simulink model "F16_model_propulsion_og"  (R2025b)
settings: Solver=VariableStepAuto  StartTime=0.0  StopTime=10.0  RelTol=1e-3
values from neighbouring files (symbols this model uses):
  b = 9.144    [initialization.m]
  c_bar = 3.45    [initialization.m]
  g = 9.81    [initialization.m]
  I = [Ixx 0 -Ixz; 0 Iyy 0; -Ixz 0 Izz]    [initialization.m]
  S = 27.87    [initialization.m]
  xcg = 0.3*c_bar    (= 1.035)    [initialization.m]
  xcgr = 0.35*c_bar    (= 1.2075)    [initialization.m]
undefined symbols (not defined in the file or in its folder): aero_data
libraries: simulink_extras x2, matrix_library x2
(part 1 of 2)
settings Model: Creator=deepa  LastModifiedBy=deepa

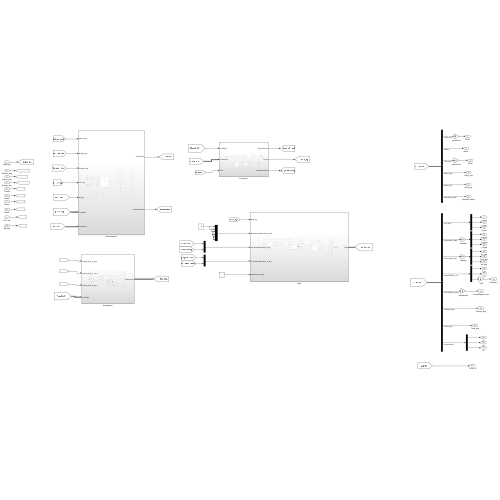
[thumbnail: Simulink's stored preview of the top-level diagram]
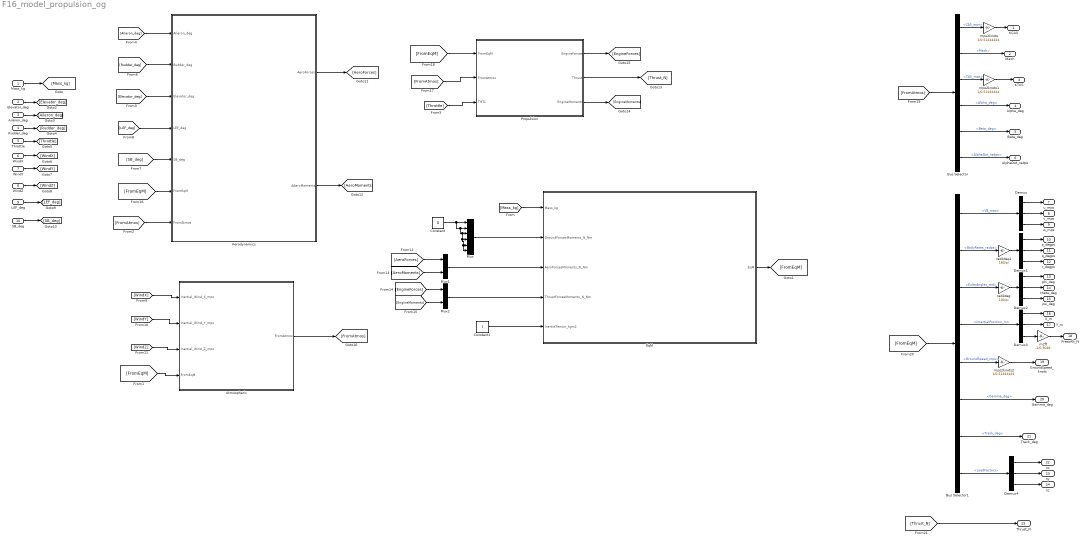
== system F16_model_propulsion_og ==
  Mass_kg : Inport  OutDataTypeStr=double
  Elevator_deg : Inport  Port=2  OutDataTypeStr=double
  Aileron_deg : Inport  Port=3  OutDataTypeStr=double
  Rudder_deg : Inport  Port=4  OutDataTypeStr=double
  Throttle : Inport  Port=5  OutDataTypeStr=double
  WindX : Inport  Port=6  OutDataTypeStr=double
  WindY : Inport  Port=7  OutDataTypeStr=double
  WindZ : Inport  Port=8  OutDataTypeStr=double
  LEF_deg : Inport  Port=9
  SB_deg : Inport  Port=10
  Aerodynamics : Subsystem
  Atmospheric : Subsystem
  Bus Selector : BusSelector  OutputSignals=CAS_mps,Mach,TAS_mps,Alpha_deg,Beta_deg,AlphaDot_radps
  Bus Selector1 : BusSelector  OutputSignals=VB_mps,BodyRates_radps,EulerAngles_rad,IntertialPosition_m,GroundSpeed_mps,Gamma_deg,Track_deg,LoadFactors
  Constant : Constant  Value=0
  Constant1 : Constant  Value=I
  Demux{,1..4} (5 alike) : Demux  Outputs=3
  EqM : Subsystem
  Mux : Mux  Inputs=6
  Mux1 : Mux  Inputs=2
  Mux2 : Mux  Inputs=2
  Propulsion : Subsystem
  m2ft : Gain  Gain=-1/0.3048
  mps2knots : Gain  Gain=1/0.51444444
  mps2knots1 : Gain  Gain=1/0.51444444
  mps2knots2 : Gain  Gain=1/0.51444444
  rad2deg : Gain  Gain=180/pi
  rad2deg1 : Gain  Gain=180/pi
  KCAS : Outport
  Mach : Outport  Port=2
  KTAS : Outport  Port=3
  Alpha_deg : Outport  Port=4
  Beta_deg : Outport  Port=5
  AlphaDot_radps : Outport  Port=6
  u_mps : Outport  Port=7
  v_mps : Outport  Port=8
  w_mps : Outport  Port=9
  p_degps : Outport  Port=10
  q_degps : Outport  Port=11
  r_degps : Outport  Port=12
  phi_deg : Outport  Port=13
  theta_deg : Outport  Port=14
  psi_deg : Outport  Port=15
  X_m : Outport  Port=16
  Y_m : Outport  Port=17
  PressAlt_ft : Outport  Port=18
  GroundSpeed_knots : Outport  Port=19
  Gamma_deg : Outport  Port=20
  Track_deg : Outport  Port=21
  nx : Outport  Port=22
  ny : Outport  Port=23
  nz : Outport  Port=24
  Thrust_N : Outport  Port=25
  wires:
  [FromAtmos] -> Propulsion/2(FromAtmos)
  Propulsion/2(Thrust) -> [Thrust_N]
  Mux/1 -> EqM/2(GroundForcesMoments_N_Nm)
  [FromEqM] -> Bus Selector1/1
  [EngineForces] -> Mux2/1
  Demux/3 -> w_mps/1
  Demux2/1 -> phi_deg/1
  [WindZ] -> Atmospheric/3(Inertial_Wind_Z_mps)
  Bus Selector1/3 -> rad2deg/1  "<EulerAngles_rad>"
  Demux1/3 -> r_degps/1
  [AeroMoments] -> Mux1/2
  LEF_deg/1 -> [LEF_deg]
  Mass_kg/1 -> [Mass_kg]
  Bus Selector1/5 -> mps2knots2/1  "<GroundSpeed_mps>"
  Bus Selector/2 -> Mach/1  "<Mach>"
  EqM/1(EqM) -> [FromEqM]
  rad2deg/1 -> Demux2/1
  Bus Selector/6 -> AlphaDot_radps/1  "<AlphaDot_radps>"
  Demux3/1 -> X_m/1
  [FromAtmos] -> Aerodynamics/7(FromAtmos)
  [Thrust_N] -> Thrust_N/1
  Demux2/3 -> psi_deg/1
  Throttle/1 -> [Throttle]
  Demux2/2 -> theta_deg/1
  Demux3/2 -> Y_m/1
  [EngineMoments] -> Mux2/2
  Demux4/2 -> ny/1
  Demux/2 -> v_mps/1
  Demux/1 -> u_mps/1
  Bus Selector/4 -> Alpha_deg/1  "<Alpha_deg>"
  [AeroForces] -> Mux1/1
  Demux4/3 -> nz/1
  [Rudder_deg] -> Aerodynamics/2(Rudder_deg)
  Elevator_deg/1 -> [Elevator_deg]
  Atmospheric/1(FromAtmos) -> [FromAtmos]
  Aerodynamics/2(AAeroMoments) -> [AeroMoments]
  Bus Selector/1 -> mps2knots/1  "<CAS_mps>"
  mps2knots/1 -> KCAS/1
  WindZ/1 -> [WindZ]
  Demux1/1 -> p_degps/1
  [SB_deg] -> Aerodynamics/5(SB_deg)
  rad2deg1/1 -> Demux1/1
  [FromAtmos] -> Bus Selector/1
  [FromEqM] -> Aerodynamics/6(FromEqM)
  [LEF_deg] -> Aerodynamics/4(LEF_deg)
  [Mass_kg] -> EqM/1(Mass_kg)
  WindX/1 -> [WindX]
  [WindX] -> Atmospheric/1(Inertial_Wind_X_mps)
  Demux4/1 -> nx/1
  Mux1/1 -> EqM/3(AeroForcesMoments_N_Nm)
  Bus Selector1/8 -> Demux4/1  "<LoadFactors>"
  mps2knots2/1 -> GroundSpeed_knots/1
  m2ft/1 -> PressAlt_ft/1
  Constant/1 -> Mux/1, Mux/6, Mux/5, Mux/4, Mux/3, Mux/2
  [Aileron_deg] -> Aerodynamics/1(Aileron_deg)
  Bus Selector1/4 -> Demux3/1  "<IntertialPosition_m>"
  Bus Selector1/7 -> Track_deg/1  "<Track_deg>"
  Mux2/1 -> EqM/4(ThrustForcesMoments_N_Nm)
  Demux1/2 -> q_degps/1
  Demux3/3 -> m2ft/1
  Constant1/1 -> EqM/5(InertiaTensor_kgm2)
  Bus Selector1/2 -> rad2deg1/1  "<BodyRates_radps>"
  Rudder_deg/1 -> [Rudder_deg]
  [WindY] -> Atmospheric/2(Inertial_Wind_Y_mps)
  Aileron_deg/1 -> [Aileron_deg]
  [Elevator_deg] -> Aerodynamics/3(Elevator_deg)
  Bus Selector/5 -> Beta_deg/1  "<Beta_deg>"
  Bus Selector/3 -> mps2knots1/1  "<TAS_mps>"
  SB_deg/1 -> [SB_deg]
  Bus Selector1/1 -> Demux/1  "<VB_mps>"
  Aerodynamics/1(AeroForces) -> [AeroForces]
  WindY/1 -> [WindY]
  [FromEqM] -> Atmospheric/4(FromEqM)
  Bus Selector1/6 -> Gamma_deg/1  "<Gamma_deg>"
  mps2knots1/1 -> KTAS/1
  [Throttle] -> Propulsion/3(THTL)
  [FromEqM] -> Propulsion/1(FromEqM)
  Propulsion/1(EngineForces) -> [EngineForces]
  Propulsion/3(EngineMoments) -> [EngineMoments]

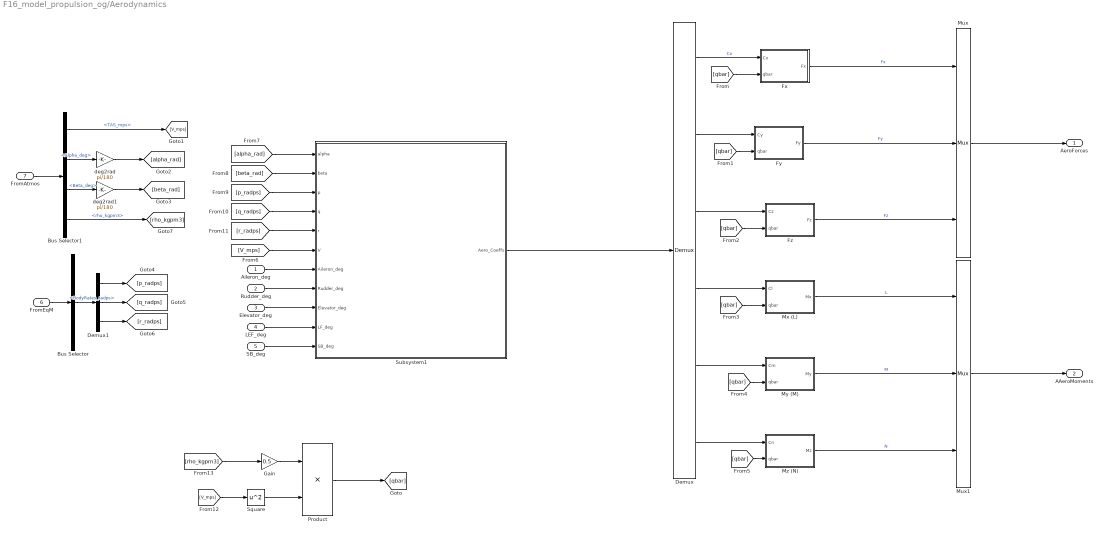
== system F16_model_propulsion_og/Aerodynamics ==
  Aileron_deg : Inport
  Rudder_deg : Inport  Port=2
  Elevator_deg : Inport  Port=3
  LEF_deg : Inport  Port=4
  SB_deg : Inport  Port=5
  FromEqM : Inport  Port=6
  FromAtmos : Inport  Port=7
  Bus Selector : BusSelector  OutputSignals=BodyRates_radps
  Bus Selector1 : BusSelector  OutputSignals=TAS_mps,Alpha_deg,Beta_deg,rho_kgpm3
  Demux : Demux  Outputs=6
  Demux1 : Demux  Outputs=3
  Fx : Subsystem
  Fy : Subsystem
  Fz : Subsystem
  Gain : Gain  Gain=0.5
  Mux : Mux  Inputs=3
  Mux1 : Mux  Inputs=3
  Mx (L) : Subsystem
  My (M) : Subsystem
  Mz (N) : Subsystem
  Product : Product
  Square : Math  Operator=square
  Subsystem1 : Subsystem
  deg2rad : Gain  Gain=pi/180
  deg2rad1 : Gain  Gain=pi/180
  AeroForces : Outport
  AAeroMoments : Outport  Port=2
  wires:
  [qbar] -> Mz (N)/2(qbar)
  Fx/1(Fx) -> Mux/1  "Fx"
  My (M)/1(My) -> Mux1/2  "M"
  [qbar] -> Fz/2(qbar)
  Fy/1(Fy) -> Mux/2  "Fy"
  Aileron_deg/1 -> Subsystem1/7(Aileron_deg)
  [qbar] -> Fx/2(qbar)
  Mux/1 -> AeroForces/1
  Subsystem1/1(Aero_Coeffs) -> Demux/1
  Fz/1(Fz) -> Mux/3  "Fz"
  [qbar] -> Fy/2(qbar)
  Demux/2 -> Fy/1(Cy)
  [p_radps] -> Subsystem1/3(p)
  [beta_rad] -> Subsystem1/2(beta)
  Demux/1 -> Fx/1(Cx)  "Cx"
  [V_mps] -> Subsystem1/6(V)
  [qbar] -> Mx (L)/2(qbar)
  [qbar] -> My (M)/2(qbar)
  Demux/4 -> Mx (L)/1(Cl)
  [alpha_rad] -> Subsystem1/1(alpha)
  Demux/6 -> Mz (N)/1(Cn)
  Demux/5 -> My (M)/1(Cm)
  Mz (N)/1(Mz) -> Mux1/3  "N"
  Mx (L)/1(Mx) -> Mux1/1  "L"
  Demux/3 -> Fz/1(Cz)
  Mux1/1 -> AAeroMoments/1
  [r_radps] -> Subsystem1/5(r)
  [q_radps] -> Subsystem1/4(q)
  Rudder_deg/1 -> Subsystem1/8(Rudder_deg)
  SB_deg/1 -> Subsystem1/11(SB_deg)
  LEF_deg/1 -> Subsystem1/10(LF_deg)
  Elevator_deg/1 -> Subsystem1/9(Elevator_deg)
  FromEqM/1 -> Bus Selector/1
  FromAtmos/1 -> Bus Selector1/1
  Bus Selector1/1 -> [V_mps]  "<TAS_mps>"
  Bus Selector1/2 -> deg2rad/1  "<Alpha_deg>"
  Bus Selector1/3 -> deg2rad1/1  "<Beta_deg>"
  deg2rad/1 -> [alpha_rad]
  deg2rad1/1 -> [beta_rad]
  Bus Selector/1 -> Demux1/1  "<BodyRates_radps>"
  Demux1/1 -> [p_radps]
  Demux1/2 -> [q_radps]
  Demux1/3 -> [r_radps]
  Bus Selector1/4 -> [rho_kgpm3]  "<rho_kgpm3>"
  [V_mps] -> Square/1
  Square/1 -> Product/2
  [rho_kgpm3] -> Gain/1
  Gain/1 -> Product/1
  Product/1 -> [qbar]

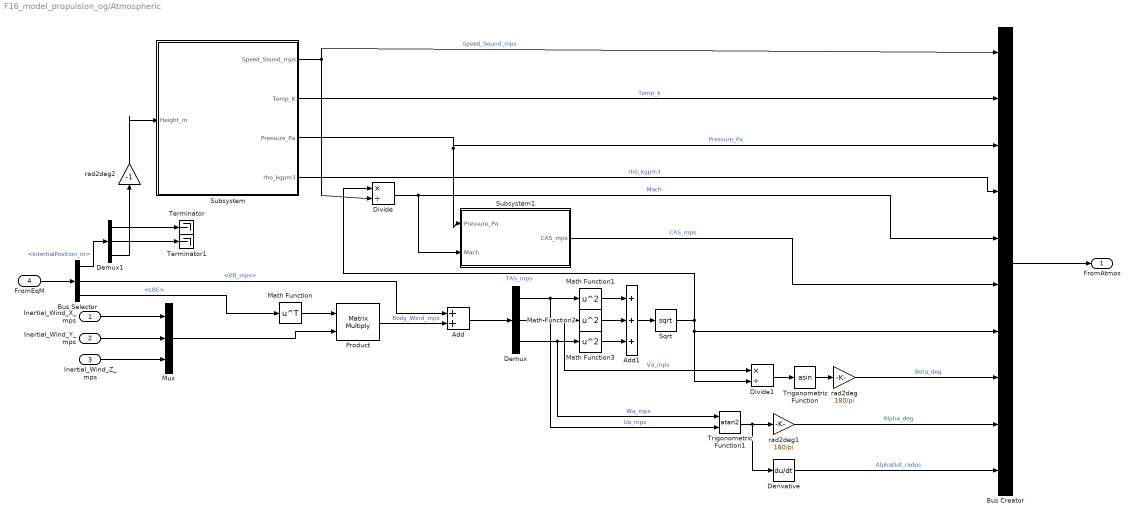
== system F16_model_propulsion_og/Atmospheric ==
  Inertial_Wind_X_mps : Inport
  Inertial_Wind_Y_mps : Inport  Port=2
  Inertial_Wind_Z_mps : Inport  Port=3
  FromEqM : Inport  Port=4
  Add : Sum
  Add1 : Sum  Inputs=+++
  Bus Creator : BusCreator  Inputs=10
  Bus Selector : BusSelector  OutputSignals=IntertialPosition_m,VB_mps,LBE
  Demux : Demux  Outputs=3
  Demux1 : Demux  Outputs=3
  Derivative : Derivative
  Divide : Product  Inputs=*/
  Divide1 : Product  Inputs=*/
  Math Function : Math  Operator=transpose  SignedPower=on
  Math Function1 : Math  Operator=square  SignedPower=on
  Math Function2 : Math  Operator=square  SignedPower=on
  Math Function3 : Math  Operator=square  SignedPower=on
  Mux : Mux  Inputs=3
  Product : Product  Multiplication=Matrix(*)
  Sqrt : Sqrt
  Subsystem : Subsystem
  Subsystem1 : Subsystem
  Terminator : Terminator
  Terminator1 : Terminator
  Trigonometric Function : Trigonometry  Operator=asin
  Trigonometric Function1 : Trigonometry  Operator=atan2
  rad2deg : Gain  Gain=180/pi
  rad2deg1 : Gain  Gain=180/pi
  rad2deg2 : Gain  Gain=-1
  FromAtmos : Outport
  wires:
  Inertial_Wind_Y_mps/1 -> Mux/2
  Demux/3 -> Math Function3/1, Trigonometric Function1/1  "Wa_mps"
  Bus Selector/1 -> Demux1/1  "<IntertialPosition_m>"
  Mux/1 -> Product/2
  Demux/1 -> Math Function1/1, Trigonometric Function1/2  "Ua_mps"
  rad2deg1/1 -> Bus Creator/9  "Alpha_deg"
  Subsystem/2(Temp_K) -> Bus Creator/2  "Temp_k"
  Bus Selector/3 -> Math Function/1  "<LBE>"
  Trigonometric Function/1 -> rad2deg/1
  rad2deg/1 -> Bus Creator/8  "Beta_deg"
  Subsystem/4(rho_kgpm3) -> Bus Creator/4  "rho_kgpm3"
  Bus Creator/1 -> FromAtmos/1
  Subsystem/3(Pressure_Pa) -> Subsystem1/1(Pressure_Pa), Bus Creator/3  "Pressure_Pa"
  Demux/2 -> Math Function2/1, Divide1/1  "Va_mps"
  Subsystem1/1(CAS_mps) -> Bus Creator/6  "CAS_mps"
  Demux1/2 -> Terminator1/1
  Divide1/1 -> Trigonometric Function/1
  Subsystem/1(Speed_Sound_mps) -> Divide/2, Bus Creator/1  "Speed_Sound_mps"
  Divide/1 -> Subsystem1/2(Mach), Bus Creator/5  "Mach"
  Demux1/1 -> Terminator/1
  Math Function2/1 -> Add1/2
  Add/1 -> Demux/1
  Derivative/1 -> Bus Creator/10  "AlphaDot_radps"
  Math Function/1 -> Product/1
  Math Function1/1 -> Add1/1
  Bus Selector/2 -> Add/1  "<VB_mps>"
  Inertial_Wind_X_mps/1 -> Mux/1
  Sqrt/1 -> Divide/1, Bus Creator/7, Divide1/2  "TAS_mps"
  FromEqM/1 -> Bus Selector/1
  Trigonometric Function1/1 -> rad2deg1/1, Derivative/1
  Inertial_Wind_Z_mps/1 -> Mux/3
  Product/1 -> Add/2  "Body_Wind_mps"
  rad2deg2/1 -> Subsystem/1("Height_m ")
  Demux1/3 -> rad2deg2/1
  Add1/1 -> Sqrt/1
  Math Function3/1 -> Add1/3

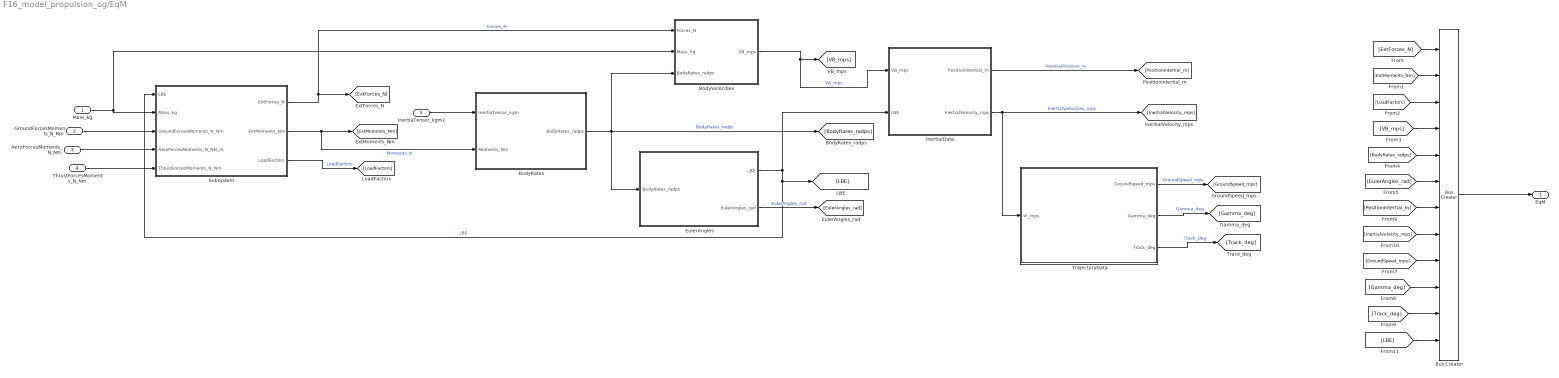
== system F16_model_propulsion_og/EqM ==
  Mass_kg : Inport
  GroundForcesMoments_N_Nm : Inport  Port=2
  AeroForcesMoments_N_Nm : Inport  Port=3
  ThrustForcesMoments_N_Nm : Inport  Port=4
  InertiaTensor_kgm2 : Inport  Port=5
  BodyRates : Subsystem
  BodyVelocities : Subsystem
  Bus Creator : BusCreator  Inputs=12
  EulerAngles : Subsystem
  InertialData : Subsystem
  Subsystem : Subsystem
  TrajectoryData : Subsystem
  EqM : Outport
  wires:
  InertiaTensor_kgm2/1 -> BodyRates/1(InertiaTensor_kgm)
  BodyRates/1(BodyRates_radps) -> EulerAngles/1(BodyRates_radps), BodyVelocities/3(BodyRates_radps), [BodyRates_radps]  "BodyRates_radps"
  AeroForcesMoments_N_Nm/1 -> Subsystem/4(AeroForcesMoments_N_NN_m)
  InertialData/1(PositionIntertial_m) -> [PositionIntertial_m]  "IntertialPosition_m"
  [GroundSpeed_mps] -> Bus Creator/9
  [PositionIntertial_m] -> Bus Creator/7
  TrajectoryData/1(GroundSpeed_mps) -> [GroundSpeed_mps]  "GroundSpeed_mps"
  Subsystem/2(ExtMoments_Nm) -> BodyRates/2(Moments_Nm), [ExtMoments_Nm]  "Moments_N"
  InertialData/2(InertialVelocity_mps) -> TrajectoryData/1(VI_mps), [InertialVelocity_mps]  "InertialVelocities_mps"
  [Track_deg] -> Bus Creator/11
  Subsystem/1(ExtForces_N) -> BodyVelocities/1(Forces_N), [ExtForces_N]  "Forces_N"
  [VB_mps] -> Bus Creator/4
  [LoadFactors] -> Bus Creator/3
  BodyVelocities/1(VB_mps) -> InertialData/1(VB_mps), [VB_mps]  "VB_mps"
  EulerAngles/2(EulerAngles_rad) -> [EulerAngles_rad]  "EulerAngles_rad"
  TrajectoryData/3(Track_deg) -> [Track_deg]  "Track_deg"
  EulerAngles/1(LBE) -> InertialData/2(LBE), Subsystem/1(LBE), [LBE]  "LBE"
  TrajectoryData/2(Gamma_deg) -> [Gamma_deg]  "Gamma_deg"
  [BodyRates_radps] -> Bus Creator/5
  [Gamma_deg] -> Bus Creator/10
  [LBE] -> Bus Creator/12
  Subsystem/3(LoadFactors) -> [LoadFactors]  "LoadFactors"
  [EulerAngles_rad] -> Bus Creator/6
  [InertialVelocity_mps] -> Bus Creator/8
  ThrustForcesMoments_N_Nm/1 -> Subsystem/5(ThrustForcesMoments_N_Nm)
  GroundForcesMoments_N_Nm/1 -> Subsystem/3(GroundForcesMoments_N_Nm)
  Bus Creator/1 -> EqM/1
  [ExtMoments_Nm] -> Bus Creator/2
  [ExtForces_N] -> Bus Creator/1
  Mass_kg/1 -> BodyVelocities/2(Mass_kg), Subsystem/2(Mass_kg)

== system F16_model_propulsion_og/Propulsion ==
  FromEqM : Inport
  FromAtmos : Inport  Port=2
  THTL : Inport  Port=3
  Bus Selector : BusSelector  OutputSignals=IntertialPosition_m
  Bus Selector1 : BusSelector  OutputSignals=Mach
  Gain : Gain  Gain=-1
  Integrator : Integrator  ContinuousStateAttributes='POW'
  Mux : Mux  Inputs=3
  Mux1 : Mux  Inputs=3
  PDOT : MATLAB Function  TreatAsAtomicUnit=on
  Selector : Selector  InputPortWidth=3  IndexOptions=Index vector (dialog)  Indices=[3]  OutputSizes=1
  TGEAR : MATLAB Function  TreatAsAtomicUnit=on
  Thrust_ : MATLAB Function  TreatAsAtomicUnit=on
  Zero : Constant  Value=0  OutDataTypeStr=Inherit: Inherit via back propagation
  Zero1 : Constant  Value=0  OutDataTypeStr=Inherit: Inherit via back propagation
  EngineForces : Outport
  Thrust : Outport  Port=2
  EngineMoments : Outport  Port=3
  wires:
  FromEqM/1 -> Bus Selector/1
  TGEAR/1(TGEAR) -> PDOT/2(P1)
  THTL/1 -> TGEAR/1(THTL)
  Mux/1 -> EngineMoments/1
  Bus Selector1/1 -> Thrust_/3(MACH)  "<Mach>"
  Thrust_/1(THRUST) -> Thrust/1, Mux1/1
  Gain/1 -> Thrust_/2(ALT)
  FromAtmos/1 -> Bus Selector1/1
  Bus Selector/1 -> Selector/1  "<IntertialPosition_m>"
  Zero/1 -> Mux/1, Mux/3, Mux/2
  Mux1/1 -> EngineForces/1
  PDOT/1(PDOT) -> Integrator/1  "Pdot"
  Zero1/1 -> Mux1/2, Mux1/3
  Integrator/1 -> PDOT/1(P3), Thrust_/1(POW)
  Selector/1 -> Gain/1

== system F16_model_propulsion_og/Aerodynamics/Fx ==
  Cx : Inport
  qbar : Inport  Port=2
  Gain : Gain  Gain=S
  Product : Product
  Fx : Outport
  wires:
  Product/1 -> Fx/1
  Gain/1 -> Product/1
  qbar/1 -> Product/2
  Cx/1 -> Gain/1

== system F16_model_propulsion_og/Aerodynamics/Fy ==
  Cy : Inport
  qbar : Inport  Port=2
  Gain : Gain  Gain=S
  Product : Product
  Fy : Outport
  wires:
  Cy/1 -> Gain/1
  qbar/1 -> Product/2
  Gain/1 -> Product/1
  Product/1 -> Fy/1

== system F16_model_propulsion_og/Aerodynamics/Fz ==
  Cz : Inport
  qbar : Inport  Port=2
  Gain : Gain  Gain=S
  Product : Product
  Fz : Outport
  wires:
  Product/1 -> Fz/1
  Gain/1 -> Product/1
  qbar/1 -> Product/2
  Cz/1 -> Gain/1

== system F16_model_propulsion_og/Aerodynamics/Mx (L) ==
  Cl : Inport
  qbar : Inport  Port=2
  Gain : Gain  Gain=S*b
  Product : Product
  Mx : Outport
  wires:
  Cl/1 -> Gain/1
  qbar/1 -> Product/2
  Gain/1 -> Product/1
  Product/1 -> Mx/1

== system F16_model_propulsion_og/Aerodynamics/My (M) ==
  Cm : Inport
  qbar : Inport  Port=2
  Gain : Gain  Gain=S*c_bar
  Product : Product
  My : Outport
  wires:
  Product/1 -> My/1
  Gain/1 -> Product/1
  qbar/1 -> Product/2
  Cm/1 -> Gain/1

== system F16_model_propulsion_og/Aerodynamics/Mz (N) ==
  Cn : Inport
  qbar : Inport  Port=2
  Gain : Gain  Gain=S*b
  Product : Product
  Mz : Outport
  wires:
  Cn/1 -> Gain/1
  qbar/1 -> Product/2
  Gain/1 -> Product/1
  Product/1 -> Mz/1

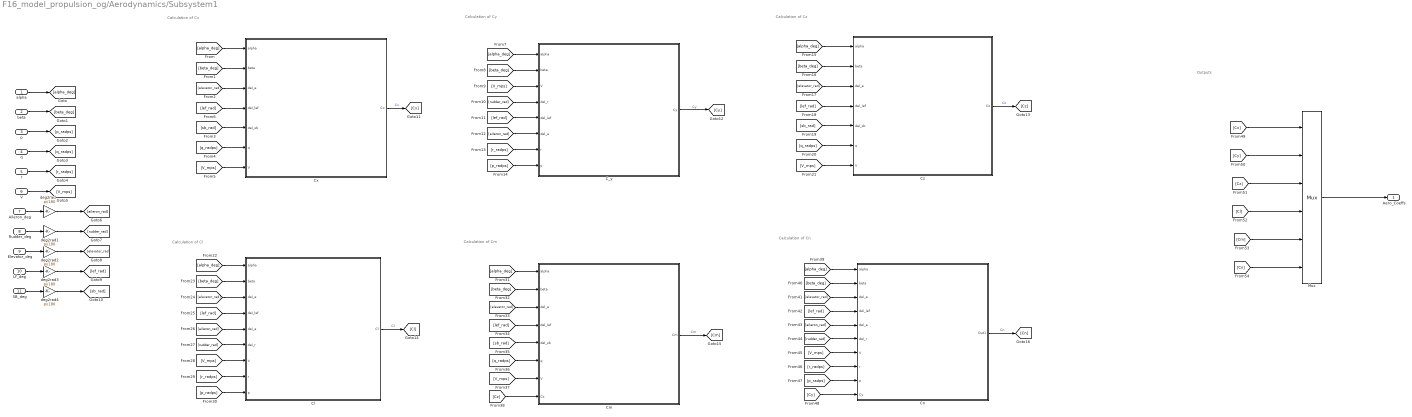
== system F16_model_propulsion_og/Aerodynamics/Subsystem1 ==
  note: Calculation of Cm
  note: Outputs
  note: Calculation of Cz
  note: Calculation of Cy
  note: Calculation of Cx
  note: Calculation of Cl
  note: Calculation of Cn
  alpha : Inport
  beta : Inport  Port=2
  p : Inport  Port=3
  q : Inport  Port=4
  r : Inport  Port=5
  V : Inport  Port=6
  Aileron_deg : Inport  Port=7
  Rudder_deg : Inport  Port=8
  Elevator_deg : Inport  Port=9
  LF_deg : Inport  Port=10
  SB_deg : Inport  Port=11
  C_y : Subsystem
  Cl : Subsystem
  Cm : Subsystem
  Cn : Subsystem
  Cx : Subsystem
  Cz : Subsystem
  Mux : Mux  Inputs=6
  deg2rad{,1..4} (5 alike) : Gain  Gain=pi/180
  Aero_Coeffs : Outport
  wires:
  V/1 -> [V_mps]
  [lef_rad] -> C_y/5(del_lef)
  [Cz] -> Mux/3
  [alpha_deg] -> C_y/1(alpha)
  [q_radps] -> Cx/6(q)
  [V_mps] -> C_y/3(V)
  alpha/1 -> [alpha_deg]
  [elevator_rad] -> Cm/3(del_e)
  Cx/1(Cx) -> [Cx]  "Cx"
  [elevator_rad] -> Cz/3(del_e)
  [rudder_rad] -> Cn/6(del_r)
  [r_radps] -> Cn/8(r)
  [beta_deg] -> C_y/2(beta)
  [elevator_rad] -> Cx/3(del_e)
  [lef_rad] -> Cx/4(del_lef)
  [Cl] -> Mux/4
  [alpha_deg] -> Cx/1(alpha)
  [alpha_deg] -> Cn/1(alpha)
  [p_radps] -> Cn/9(p)
  r/1 -> [r_radps]
  Cl/1(Cl) -> [Cl]  "Cl"
  C_y/1(Cy) -> [Cy]  "Cy"
  Cz/1(Cz) -> [Cz]  "Cz"
  [r_radps] -> Cl/8(r)
  SB_deg/1 -> deg2rad4/1
  LF_deg/1 -> deg2rad3/1
  [elevator_rad] -> Cn/3(del_e)
  [beta_deg] -> Cm/2(beta)
  [p_radps] -> C_y/8(p)
  [q_radps] -> Cm/6(q)
  [alpha_deg] -> Cz/1(alpha)
  [V_mps] -> Cl/7(V)
  [alpha_deg] -> Cl/1(alpha)
  [beta_deg] -> Cl/2(beta)
  [lef_rad] -> Cz/4(del_lef)
  Mux/1 -> Aero_Coeffs/1
  [alpha_deg] -> Cm/1(alpha)
  [V_mps] -> Cm/7(V)
  beta/1 -> [beta_deg]
  Rudder_deg/1 -> deg2rad1/1
  [sb_rad] -> Cz/5(del_sb)
  [sb_rad] -> Cx/5(del_sb)
  [Cy] -> Mux/2
  [rudder_rad] -> C_y/4(del_r)
  Aileron_deg/1 -> deg2rad/1
  [beta_deg] -> Cz/2(beta)
  [Cz] -> Cm/8(Cz)
  [V_mps] -> Cz/7(V)
  [V_mps] -> Cn/7(V)
  [r_radps] -> C_y/7(r)
  [lef_rad] -> Cl/4(del_lef)
  [sb_rad] -> Cm/5(del_sb)
  [q_radps] -> Cz/6(q)
  [Cm] -> Mux/5
  Elevator_deg/1 -> deg2rad2/1
  q/1 -> [q_radps]
  [aileron_rad] -> Cn/5(del_a)
  [p_radps] -> Cl/9(p)
  [rudder_rad] -> Cl/6(del_r)
  [elevator_rad] -> Cl/3(del_e)
  p/1 -> [p_radps]
  [aileron_rad] -> Cl/5(del_a)
  [Cn] -> Mux/6
  [lef_rad] -> Cm/4(del_lef)
  [beta_deg] -> Cn/2(beta)
  [Cy] -> Cn/10(Cy)
  [aileron_rad] -> C_y/6(del_a)
  [V_mps] -> Cx/7(V)
  Cn/1(Out1) -> [Cn]  "Cn"
  [beta_deg] -> Cx/2(beta)
  [lef_rad] -> Cn/4(del_lef)
  [Cx] -> Mux/1
  Cm/1(Cm) -> [Cm]  "Cm"
  deg2rad/1 -> [aileron_rad]
  deg2rad1/1 -> [rudder_rad]
  deg2rad2/1 -> [elevator_rad]
  deg2rad3/1 -> [lef_rad]
  deg2rad4/1 -> [sb_rad]

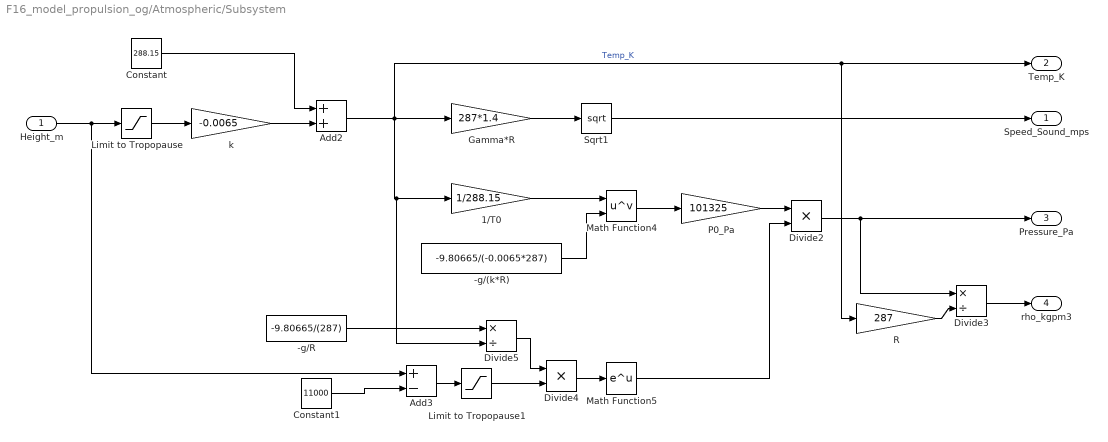
== system F16_model_propulsion_og/Atmospheric/Subsystem ==
  "Height_m " : Inport
  -g/(k*R) : Constant  Value=-9.80665/(-0.0065*287)
  -g/R : Constant  Value=-9.80665/(287)
  1/T0 : Gain  Gain=1/288.15
  Add2 : Sum
  Add3 : Sum  Inputs=+-
  Constant : Constant  Value=288.15
  Constant1 : Constant  Value=11000
  Divide2 : Product  Inputs=**
  Divide3 : Product  Inputs=*/
  Divide4 : Product  Inputs=**
  Divide5 : Product  Inputs=*/
  Gamma*R : Gain  Gain=287*1.4
  Limit to Tropopause : Saturate  UpperLimit=11000  LowerLimit=0
  Limit to Tropopause1 : Saturate  UpperLimit=inf  LowerLimit=0
  Math Function4 : Math  Operator=pow  SignedPower=on
  Math Function5 : Math  SignedPower=on
  P0_Pa : Gain  Gain=101325
  R : Gain  Gain=287
  Sqrt1 : Sqrt
  k : Gain  Gain=-0.0065
  Speed_Sound_mps : Outport
  Temp_K : Outport  Port=2
  Pressure_Pa : Outport  Port=3
  rho_kgpm3 : Outport  Port=4
  wires:
  Add3/1 -> Limit to Tropopause1/1
  Divide5/1 -> Divide4/1
  1/T0/1 -> Math Function4/1
  Add2/1 -> Divide5/2, 1/T0/1, Temp_K/1, R/1, Gamma*R/1  "Temp_K"
  Limit to Tropopause/1 -> k/1
  Limit to Tropopause1/1 -> Divide4/2
  Divide2/1 -> Pressure_Pa/1, Divide3/1
  Divide4/1 -> Math Function5/1
  R/1 -> Divide3/2
  -g/(k*R)/1 -> Math Function4/2
  Constant1/1 -> Add3/2
  "Height_m "/1 -> Add3/1, Limit to Tropopause/1
  Constant/1 -> Add2/1
  Divide3/1 -> rho_kgpm3/1
  Gamma*R/1 -> Sqrt1/1
  k/1 -> Add2/2
  -g/R/1 -> Divide5/1
  Sqrt1/1 -> Speed_Sound_mps/1
  Math Function5/1 -> Divide2/2
  Math Function4/1 -> P0_Pa/1
  P0_Pa/1 -> Divide2/1

== system F16_model_propulsion_og/Atmospheric/Subsystem1 ==
  Pressure_Pa : Inport
  Mach : Inport  Port=2
  (Gamma-1)/2 : Gain  Gain=(1.4-1)/2
  (Gamma-1)/Gamma : Constant  Value=(1.4-1)/1.4
  2*a0^2/(Gamma-1) : Gain  Gain=(2*340.262^2)/(1.4-1)
  Add2 : Sum
  Add3 : Sum  Inputs=+-
  Add4 : Sum
  Add5 : Sum  Inputs=+-
  Constant2 : Constant
  Divide5 : Product  Inputs=**
  Divide6 : Product  Inputs=*/
  Gamma/(Gamma-1) : Constant  Value=1.4/(1.4-1)
  Math Function4 : Math  Operator=square  SignedPower=on
  Math Function5 : Math  Operator=pow  SignedPower=on
  Math Function6 : Math  Operator=pow  SignedPower=on
  P0_Pa : Constant  Value=101325
  Sqrt2 : Sqrt
  CAS_mps : Outport
  wires:
  Constant2/1 -> Add2/2, Add3/2, Add4/2, Add5/2
  Math Function5/1 -> Add3/1
  Gamma/(Gamma-1)/1 -> Math Function5/2
  Add5/1 -> 2*a0^2/(Gamma-1)/1
  Pressure_Pa/1 -> Divide5/1
  Add4/1 -> Math Function6/1
  P0_Pa/1 -> Divide6/2
  (Gamma-1)/Gamma/1 -> Math Function6/2
  Sqrt2/1 -> CAS_mps/1
  Divide5/1 -> Divide6/1  "pt-ps"
  Add3/1 -> Divide5/2
  Math Function6/1 -> Add5/1
  Mach/1 -> Math Function4/1
  2*a0^2/(Gamma-1)/1 -> Sqrt2/1
  Add2/1 -> Math Function5/1
  Divide6/1 -> Add4/1
  (Gamma-1)/2/1 -> Add2/1
  Math Function4/1 -> (Gamma-1)/2/1

== system F16_model_propulsion_og/EqM/BodyRates ==
  InertiaTensor_kgm : Inport
  Moments_Nm : Inport  Port=2
  Cross Product : matrix_library/Cross Product
  Demux : Demux  Outputs=3
  Divide : Product  Inputs=/*  Multiplication=Matrix(*)
  Mux : Mux  Inputs=3
  Product : Product  Multiplication=Matrix(*)
  Sum : Sum  Inputs=|-+
  p_radps : Integrator  ContinuousStateAttributes='p_radps'
  q_radps : Integrator  ContinuousStateAttributes='q_radps'
  r_radps : Integrator  ContinuousStateAttributes='r_radps'
  BodyRates_radps : Outport
  wires:
  Mux/1 -> BodyRates_radps/1, Cross Product/1, Product/2
  p_radps/1 -> Mux/1  "p_radps"
  Demux/2 -> q_radps/1
  Demux/1 -> p_radps/1
  q_radps/1 -> Mux/2  "q_radps"
  Demux/3 -> r_radps/1
  InertiaTensor_kgm/1 -> Divide/1, Product/1
  r_radps/1 -> Mux/3  "r_radps"
  Moments_Nm/1 -> Sum/2
  Divide/1 -> Demux/1
  Product/1 -> Cross Product/2
  Cross Product/1 -> Sum/1
  Sum/1 -> Divide/2

== system F16_model_propulsion_og/EqM/BodyVelocities ==
  Forces_N : Inport
  Mass_kg : Inport  Port=2
  BodyRates_radps : Inport  Port=3
  Add : Sum  Inputs=+-
  Cross Product : matrix_library/Cross Product
  Demux : Demux  Outputs=3
  Divide : Product  Inputs=*/
  Mux : Mux  Inputs=3
  u_mps : Integrator  ContinuousStateAttributes='u_mps'
  v_mps : Integrator  ContinuousStateAttributes='v_mps'
  w_mps : Integrator  ContinuousStateAttributes='w_mps'
  VB_mps : Outport
  wires:
  Demux/3 -> w_mps/1
  u_mps/1 -> Mux/1
  Add/1 -> Demux/1  "VB_dot_mps2"
  Divide/1 -> Add/1
  Mass_kg/1 -> Divide/2
  Demux/2 -> v_mps/1
  BodyRates_radps/1 -> Cross Product/1
  Mux/1 -> Cross Product/2, VB_mps/1
  w_mps/1 -> Mux/3
  Demux/1 -> u_mps/1
  v_mps/1 -> Mux/2
  Cross Product/1 -> Add/2
  Forces_N/1 -> Divide/1

== system F16_model_propulsion_og/EqM/EulerAngles ==
  BodyRates_radps : Inport
  Demux : Demux  Outputs=3
  Mux1 : Mux  Inputs=3
  PHI_rad : Integrator  ContinuousStateAttributes='PHI_rad'
  PSI_rad : Integrator  ContinuousStateAttributes='PSI_rad'
  Rotation Matrix : Subsystem
  Subsystem : Subsystem
  THETA_rad : Integrator  ContinuousStateAttributes='THETA_rad'
  LBE : Outport
  EulerAngles_rad : Outport  Port=2
  wires:
  BodyRates_radps/1 -> Subsystem/1("BodyRates_radps ")
  Subsystem/1(EulerRates_radsps2) -> Demux/1
  Mux1/1 -> Rotation Matrix/1(EulerAngles_rad), Subsystem/2(EulerAngles_rad), EulerAngles_rad/1
  Demux/1 -> PHI_rad/1
  PSI_rad/1 -> Mux1/3
  PHI_rad/1 -> Mux1/1
  Rotation Matrix/1(LBE) -> LBE/1
  Demux/3 -> PSI_rad/1
  THETA_rad/1 -> Mux1/2
  Demux/2 -> THETA_rad/1

== system F16_model_propulsion_og/EqM/InertialData ==
  VB_mps : Inport
  LBE : Inport  Port=2
  Demux : Demux  Outputs=3
  Mux : Mux  Inputs=3
  Product : Product  Multiplication=Matrix(*)
  XI_m : Integrator  ContinuousStateAttributes='XI_m'
  YI_m1 : Integrator  ContinuousStateAttributes='YI_m'
  ZI_m : Integrator  ContinuousStateAttributes='ZI_m'
  PositionIntertial_m : Outport
  InertialVelocity_mps : Outport  Port=2
  wires:
  Product/1 -> InertialVelocity_mps/1, Demux/1  "VI_mps"
  ZI_m/1 -> Mux/3
  Demux/1 -> XI_m/1
  VB_mps/1 -> Product/2
  Demux/2 -> YI_m1/1
  Mux/1 -> PositionIntertial_m/1
  YI_m1/1 -> Mux/2
  LBE/1 -> Product/1
  XI_m/1 -> Mux/1
  Demux/3 -> ZI_m/1

== system F16_model_propulsion_og/EqM/Subsystem ==
  LBE : Inport
  Mass_kg : Inport  Port=2
  GroundForcesMoments_N_Nm : Inport  Port=3
  AeroForcesMoments_N_NN_m : Inport  Port=4
  ThrustForcesMoments_N_Nm : Inport  Port=5
  Add : Sum  Inputs=+++
  Constant : Constant  Value=0
  Demux : Demux  Outputs=2
  Demux1 : Demux  Outputs=3
  Divide : Product  Inputs=*/  Multiplication=Matrix(*)
  Gain : Gain  Gain=-1
  Math Function : Math  Operator=transpose  SignedPower=on
  Mux : Mux  Inputs=3
  Mux1 : Mux  Inputs=3
  Product : Product  Multiplication=Matrix(*)
  Sum : Sum  Inputs=|++
  g_mps2 : Gain  Gain=g
  ExtForces_N : Outport
  ExtMoments_Nm : Outport  Port=2
  LoadFactors : Outport  Port=3
  wires:
  Demux/1 -> Sum/2, Divide/1  "Forces"
  Demux1/1 -> Mux1/1  "nx"
  Demux1/3 -> Gain/1
  ThrustForcesMoments_N_Nm/1 -> Add/3
  Product/1 -> Sum/1  "Weight_N_body"
  Mux/1 -> Product/2
  g_mps2/1 -> Divide/2, Mux/3  "Weight_N"
  LBE/1 -> Math Function/1
  Sum/1 -> ExtForces_N/1
  Add/1 -> Demux/1
  Math Function/1 -> Product/1  "LEB"
  Demux/2 -> ExtMoments_Nm/1  "Moments"
  Mass_kg/1 -> g_mps2/1
  Gain/1 -> Mux1/3  "nz"
  Divide/1 -> Demux1/1
  GroundForcesMoments_N_Nm/1 -> Add/1
  Constant/1 -> Mux/2, Mux/1
  Mux1/1 -> LoadFactors/1
  AeroForcesMoments_N_NN_m/1 -> Add/2
  Demux1/2 -> Mux1/2  "ny"

== system F16_model_propulsion_og/EqM/TrajectoryData ==
  VI_mps : Inport
  Add : Sum
  Demux : Demux  Outputs=3
  Gain : Gain  Gain=-1
  Gain1 : Gain  Gain=180/pi
  Gain2 : Gain  Gain=180/pi
  Math Function : Math  Operator=square  SignedPower=on
  Math Function1 : Math  Operator=square  SignedPower=on
  Sqrt : Sqrt
  Trigonometric Function : Trigonometry  Operator=atan2
  Trigonometric Function1 : Trigonometry  Operator=atan2
  GroundSpeed_mps : Outport
  Gamma_deg : Outport  Port=2
  Track_deg : Outport  Port=3
  wires:
  VI_mps/1 -> Demux/1
  Gain/1 -> Trigonometric Function/1
  Math Function/1 -> Add/1
  Sqrt/1 -> GroundSpeed_mps/1, Trigonometric Function/2
  Demux/2 -> Trigonometric Function1/1, Math Function1/1
  Trigonometric Function/1 -> Gain1/1
  Add/1 -> Sqrt/1
  Gain1/1 -> Gamma_deg/1
  Math Function1/1 -> Add/2
  Gain2/1 -> Track_deg/1
  Demux/3 -> Gain/1
  Demux/1 -> Trigonometric Function1/2, Math Function/1
  Trigonometric Function1/1 -> Gain2/1

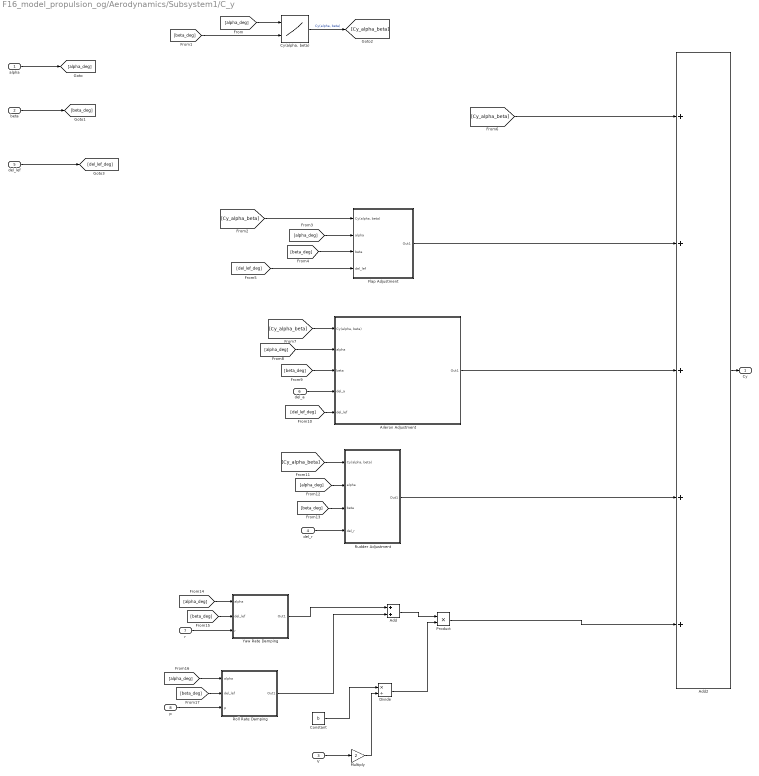
== system F16_model_propulsion_og/Aerodynamics/Subsystem1/C_y ==
  alpha : Inport
  beta : Inport  Port=2
  V : Inport  Port=3
  del_r : Inport  Port=4
  del_lef : Inport  Port=5
  del_a : Inport  Port=6
  r : Inport  Port=7
  p : Inport  Port=8
  Add : Sum
  Add2 : Sum  Inputs=+++++
  Aileron Adjustment : Subsystem
  Constant : Constant  Value=b
  "Cy(alpha, beta)" : Lookup_n-D  BreakpointsForDimension1=[-20, -15, -10, -5, 0, 5, 10, 15, 20, 25, 30, 35, 40, 45, 50, 55, 60, 70, 80, 90];  BreakpointsForDimension2=[-30, -25, -20, -15, -10, -8, -6, -4, -2, 0, 2, 4, 6, 8, 10, 15, 20, 25, 30];  Table=aero_data.Cy_alpha_beta  InternalRulePriority=Speed  RndMeth=Simplest
      settings: InputPortMap=u0,u1
  Divide : Product  Inputs=*/
  Flap Adjustment : Subsystem
  Multiply : Gain  Gain=2
  Product : Product
  Roll Rate Damping : Subsystem
  Rudder Adjustment : Subsystem
  Yaw Rate Damping : Subsystem
  Cy : Outport
  wires:
  Product/1 -> Add2/5
  Roll Rate Damping/1(Out1) -> Add/2
  Add/1 -> Product/1
  del_r/1 -> Rudder Adjustment/4(del_r)
  Yaw Rate Damping/1(Out1) -> Add/1
  p/1 -> Roll Rate Damping/3(p)
  Add2/1 -> Cy/1
  r/1 -> Yaw Rate Damping/3(r)
  del_a/1 -> Aileron Adjustment/4(del_a)
  Divide/1 -> Product/2
  Aileron Adjustment/1(Out1) -> Add2/3
  V/1 -> Multiply/1
  Flap Adjustment/1(Out1) -> Add2/2
  Rudder Adjustment/1(Out1) -> Add2/4
  Constant/1 -> Divide/1
  Multiply/1 -> Divide/2
  alpha/1 -> [alpha_deg]
  beta/1 -> [beta_deg]
  [alpha_deg] -> "Cy(alpha, beta)"/1
  [beta_deg] -> "Cy(alpha, beta)"/2
  "Cy(alpha, beta)"/1 -> [Cy_alpha_beta]  "Cy(alpha, beta)"
  [Cy_alpha_beta] -> Flap Adjustment/1("Cy(alpha, beta)")
  [alpha_deg] -> Flap Adjustment/2(alpha)
  [beta_deg] -> Flap Adjustment/3(beta)
  del_lef/1 -> [del_lef_deg]
  [del_lef_deg] -> Flap Adjustment/4(del_lef)
  [Cy_alpha_beta] -> Add2/1
  [Cy_alpha_beta] -> Aileron Adjustment/1("Cy(alpha, beta)")
  [alpha_deg] -> Aileron Adjustment/2(alpha)
  [beta_deg] -> Aileron Adjustment/3(beta)
  [del_lef_deg] -> Aileron Adjustment/5(del_lef)
  [Cy_alpha_beta] -> Rudder Adjustment/1("Cy(alpha, beta)")
  [alpha_deg] -> Rudder Adjustment/2(alpha)
  [beta_deg] -> Rudder Adjustment/3(beta)
  [alpha_deg] -> Yaw Rate Damping/1(alpha)
  [beta_deg] -> Yaw Rate Damping/2(del_lef)
  [alpha_deg] -> Roll Rate Damping/1(alpha)
  [beta_deg] -> Roll Rate Damping/2(del_lef)

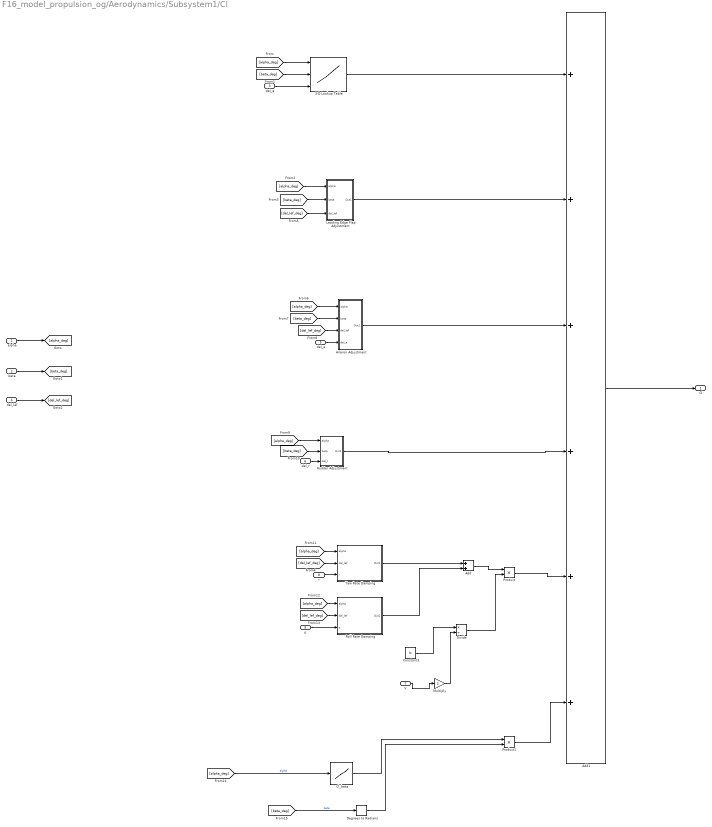
== system F16_model_propulsion_og/Aerodynamics/Subsystem1/Cl ==
  alpha : Inport
  beta : Inport  Port=2
  del_e : Inport  Port=3
  del_lef : Inport  Port=4
  del_a : Inport  Port=5
  del_r : Inport  Port=6
  V : Inport  Port=7
  r : Inport  Port=8
  p : Inport  Port=9
  3-D Lookup Table : Lookup_n-D  NumberOfTableDimensions=3  BreakpointsForDimension1=[-20, -15, -10, -5, 0, 5, 10, 15, 20, 25, 30, 35, 40, 45, 50, 55, 60, 70, 80, 90];  BreakpointsForDimension2=[-30, -25, -20, -15, -10, -8, -6, -4, -2, 0, 2, 4, 6, 8, 10, 15, 20, 25, 30];  BreakpointsForDimension3=[-25,0,25];  Table=aero_data.Cl_del_h  InternalRulePriority=Speed  RndMeth=Simplest
      settings: InputPortMap=u0,u1,u2
  Add : Sum
  Add1 : Sum  Inputs=++++++
  Aileron Adjustment : Subsystem
  Cl_beta : Lookup_n-D  NumberOfTableDimensions=1  BreakpointsForDimension1=[-20, -15, -10, -5, 0, 5, 10, 15, 20, 25, 30, 35, 40, 45, 50, 55, 60, 70, 80, 90];  Table=aero_data.del_Cl_beta  InternalRulePriority=Speed  RndMeth=Simplest
  Constant3 : Constant  Value=b
  Degrees to Radians : simulink_extras/Transformations/Degrees to Radians
  Divide : Product  Inputs=*/
  Leading Edge Flap Adjustment : Subsystem
  Multiply : Gain  Gain=2
  Product : Product
  Product1 : Product
  Roll Rate Damping : Subsystem
  Rudder Adjustment : Subsystem
  Yaw Rate Damping : Subsystem
  Cl : Outport
  wires:
  r/1 -> Yaw Rate Damping/3(r)
  Roll Rate Damping/1(Out1) -> Add/2
  del_r/1 -> Rudder Adjustment/3(del_r)
  Multiply/1 -> Divide/2
  Product/1 -> Add1/5
  p/1 -> Roll Rate Damping/3(p)
  del_a/1 -> Aileron Adjustment/4(del_a)
  3-D Lookup Table/1 -> Add1/1
  Constant3/1 -> Divide/1
  Rudder Adjustment/1(Out1) -> Add1/4
  Add1/1 -> Cl/1
  Leading Edge Flap Adjustment/1(Out1) -> Add1/2
  Yaw Rate Damping/1(Out1) -> Add/1
  Add/1 -> Product/1
  V/1 -> Multiply/1
  Divide/1 -> Product/2
  Cl_beta/1 -> Product1/1
  Degrees to Radians/1 -> Product1/2
  Product1/1 -> Add1/6
  [beta_deg] -> Degrees to Radians/1  "beta"
  [alpha_deg] -> Cl_beta/1  "alpha"
  alpha/1 -> [alpha_deg]
  beta/1 -> [beta_deg]
  [alpha_deg] -> 3-D Lookup Table/1
  [beta_deg] -> 3-D Lookup Table/2
  del_e/1 -> 3-D Lookup Table/3
  [alpha_deg] -> Leading Edge Flap Adjustment/1(alpha)
  [beta_deg] -> Leading Edge Flap Adjustment/2(beta)
  del_lef/1 -> [del_lef_deg]
  [del_lef_deg] -> Yaw Rate Damping/2(del_lef)
  [del_lef_deg] -> Leading Edge Flap Adjustment/3(del_lef)
  [alpha_deg] -> Aileron Adjustment/1(alpha)
  [beta_deg] -> Aileron Adjustment/2(beta)
  [del_lef_deg] -> Aileron Adjustment/3(del_lef)
  [alpha_deg] -> Rudder Adjustment/1(alpha)
  [beta_deg] -> Rudder Adjustment/2(beta)
  [alpha_deg] -> Yaw Rate Damping/1(alpha)
  [alpha_deg] -> Roll Rate Damping/1(alpha)
  [del_lef_deg] -> Roll Rate Damping/2(del_lef)
  Aileron Adjustment/1(Out1) -> Add1/3

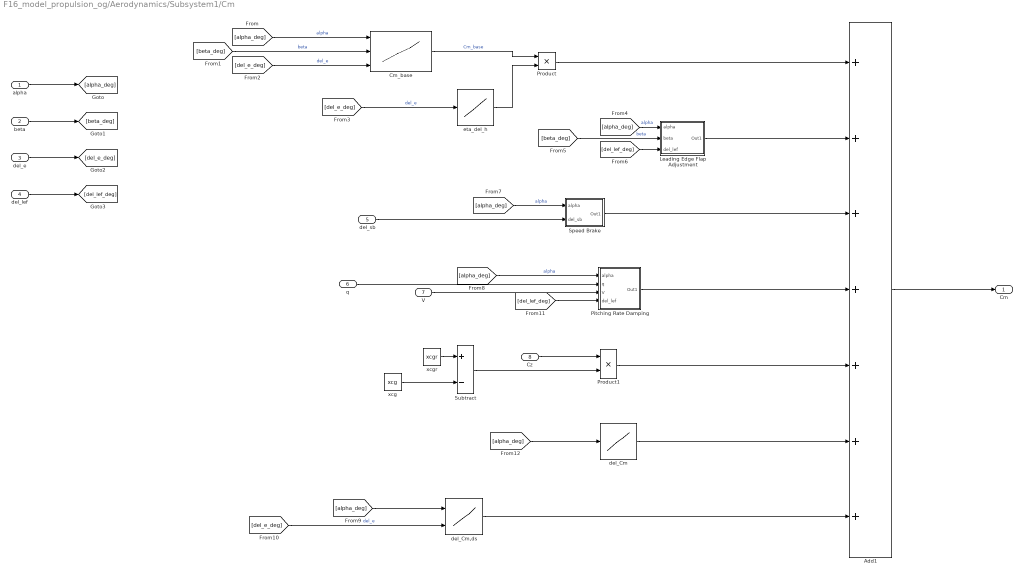
== system F16_model_propulsion_og/Aerodynamics/Subsystem1/Cm ==
  alpha : Inport
  beta : Inport  Port=2
  del_e : Inport  Port=3
  del_lef : Inport  Port=4
  del_sb : Inport  Port=5
  q : Inport  Port=6
  V : Inport  Port=7
  Cz : Inport  Port=8
  " Cm_base" : Lookup_n-D  NumberOfTableDimensions=3  BreakpointsForDimension1=[-20, -15, -10, -5, 0, 5, 10, 15, 20, 25, 30, 35, 40, 45, 50, 55, 60, 70, 80, 90];  BreakpointsForDimension2=[-30, -25, -20, -15, -10, -8, -6, -4, -2, 0, 2, 4, 6, 8, 10, 15, 20, 25, 30];  BreakpointsForDimension3=[-25, -10, 0, 10, 25]  Table=aero_data.Cm_del_h  InternalRulePriority=Speed  RndMeth=Simplest
      settings: InputPortMap=u0,u1,u2
  Add1 : Sum  Inputs=+++++++
  Leading Edge Flap Adjustment : Subsystem
  Pitching Rate Damping : Subsystem
  Product : Product
  Product1 : Product
  Speed Brake : Subsystem
  Subtract : Sum  Inputs=+-
  del_Cm : Lookup_n-D  NumberOfTableDimensions=1  BreakpointsForDimension1=[-20, -15, -10, -5, 0, 5, 10, 15, 20, 25, 30, 35, 40, 45, 50, 55, 60, 70, 80, 90]  Table=aero_data.del_Cm  InternalRulePriority=Speed  RndMeth=Simplest
  del_Cm,ds : Lookup_n-D  BreakpointsForDimension1=[-20, -15, -10, -5, 0, 5, 10, 15, 20, 25, 30, 35, 40, 45, 50, 55, 60, 70, 80, 90];  BreakpointsForDimension2=[-25, -10, 0, 10, 15, 20, 25]  Table=aero_data.del_Cm_ds  InternalRulePriority=Speed  RndMeth=Simplest
      settings: InputPortMap=u0,u1
  eta_del_h : Lookup_n-D  NumberOfTableDimensions=1  BreakpointsForDimension1=[-25, -10, 0, 10, 25]  Table=aero_data.eta_del_h  InternalRulePriority=Speed  RndMeth=Simplest
  xcg : Constant  Value=xcg
  xcgr : Constant  Value=xcgr
  Cm : Outport
  wires:
  Speed Brake/1(Out1) -> Add1/3
  Pitching Rate Damping/1(Out1) -> Add1/4
  Leading Edge Flap Adjustment/1(Out1) -> Add1/2
  Add1/1 -> Cm/1
  del_sb/1 -> Speed Brake/2(del_sb)
  q/1 -> Pitching Rate Damping/2(q)
  V/1 -> Pitching Rate Damping/3(V)
  " Cm_base"/1 -> Product/1  "Cm_base"
  eta_del_h/1 -> Product/2
  Product/1 -> Add1/1
  Cz/1 -> Product1/1
  xcgr/1 -> Subtract/1
  xcg/1 -> Subtract/2
  Subtract/1 -> Product1/2
  Product1/1 -> Add1/5
  del_Cm/1 -> Add1/6
  del_Cm,ds/1 -> Add1/7
  [alpha_deg] -> " Cm_base"/1  "alpha"
  [beta_deg] -> " Cm_base"/2  "beta"
  [del_e_deg] -> eta_del_h/1  "del_e"
  [del_e_deg] -> " Cm_base"/3  "del_e"
  alpha/1 -> [alpha_deg]
  beta/1 -> [beta_deg]
  del_e/1 -> [del_e_deg]
  del_lef/1 -> [del_lef_deg]
  [alpha_deg] -> Leading Edge Flap Adjustment/1(alpha)  "alpha"
  [beta_deg] -> Leading Edge Flap Adjustment/2(beta)  "beta"
  [del_lef_deg] -> Leading Edge Flap Adjustment/3(del_lef)
  [alpha_deg] -> Speed Brake/1(alpha)  "alpha"
  [alpha_deg] -> Pitching Rate Damping/1(alpha)  "alpha"
  [alpha_deg] -> del_Cm,ds/1
  [del_e_deg] -> del_Cm,ds/2  "del_e"
  [del_lef_deg] -> Pitching Rate Damping/4(del_lef)
  [alpha_deg] -> del_Cm/1

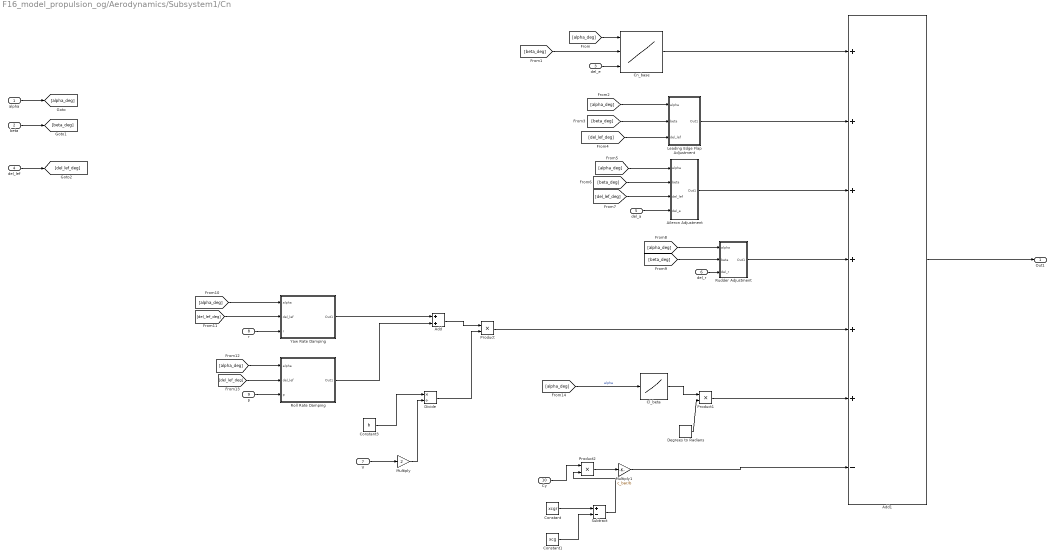
== system F16_model_propulsion_og/Aerodynamics/Subsystem1/Cn ==
  alpha : Inport
  beta : Inport  Port=2
  del_e : Inport  Port=3
  del_lef : Inport  Port=4
  del_a : Inport  Port=5
  del_r : Inport  Port=6
  V : Inport  Port=7
  r : Inport  Port=8
  p : Inport  Port=9
  Cy : Inport  Port=10
  Add : Sum
  Add1 : Sum  Inputs=++++++-
  Aileron Adjustment : Subsystem
  Cl_beta : Lookup_n-D  NumberOfTableDimensions=1  BreakpointsForDimension1=[-20, -15, -10, -5, 0, 5, 10, 15, 20, 25, 30, 35, 40, 45, 50, 55, 60, 70, 80, 90];  Table=aero_data.del_Cn_beta  InternalRulePriority=Speed  RndMeth=Simplest
  Cn_base : Lookup_n-D  NumberOfTableDimensions=3  BreakpointsForDimension1=[-20, -15, -10, -5, 0, 5, 10, 15, 20, 25, 30, 35, 40, 45, 50, 55, 60, 70, 80, 90];  BreakpointsForDimension2=[-30, -25, -20, -15, -10, -8, -6, -4, -2, 0, 2, 4, 6, 8, 10, 15, 20, 25, 30];  BreakpointsForDimension3=[-25,0,25];  Table=aero_data.Cn_del_h  InternalRulePriority=Speed  RndMeth=Simplest
      settings: InputPortMap=u0,u1,u2
  Constant : Constant  Value=xcgr
  Constant1 : Constant  Value=xcg
  Constant3 : Constant  Value=b
  Degrees to Radians : simulink_extras/Transformations/Degrees to Radians
  Divide : Product  Inputs=*/
  Leading Edge Flap Adjustment : Subsystem
  Multiply : Gain  Gain=2
  Multiply1 : Gain  Gain=c_bar/b
  Product : Product
  Product1 : Product
  Product2 : Product
  Roll Rate Damping : Subsystem
  Rudder Adjustment : Subsystem
  Subtract : Sum  Inputs=+-
  Yaw Rate Damping : Subsystem
  Out1 : Outport
  wires:
  r/1 -> Yaw Rate Damping/3(r)
  Roll Rate Damping/1(Out1) -> Add/2
  del_r/1 -> Rudder Adjustment/3(del_r)
  Aileron Adjustment/1(Out1) -> Add1/3
  Multiply/1 -> Divide/2
  Product/1 -> Add1/5
  p/1 -> Roll Rate Damping/3(p)
  del_a/1 -> Aileron Adjustment/4(del_a)
  Cn_base/1 -> Add1/1
  Constant3/1 -> Divide/1
  Rudder Adjustment/1(Out1) -> Add1/4
  Add1/1 -> Out1/1
  Leading Edge Flap Adjustment/1(Out1) -> Add1/2
  Yaw Rate Damping/1(Out1) -> Add/1
  del_e/1 -> Cn_base/3
  Add/1 -> Product/1
  V/1 -> Multiply/1
  Divide/1 -> Product/2
  Cl_beta/1 -> Product1/1
  Degrees to Radians/1 -> Product1/2
  Product1/1 -> Add1/6
  Constant/1 -> Subtract/1
  Constant1/1 -> Subtract/2
  Cy/1 -> Product2/1
  Subtract/1 -> Product2/2
  Product2/1 -> Multiply1/1
  Multiply1/1 -> Add1/7
  [alpha_deg] -> Cl_beta/1  "alpha"
  alpha/1 -> [alpha_deg]
  beta/1 -> [beta_deg]
  del_lef/1 -> [del_lef_deg]
  [alpha_deg] -> Cn_base/1
  [beta_deg] -> Cn_base/2
  [alpha_deg] -> Leading Edge Flap Adjustment/1(alpha)
  [beta_deg] -> Leading Edge Flap Adjustment/2(beta)
  [del_lef_deg] -> Leading Edge Flap Adjustment/3(del_lef)
  [alpha_deg] -> Aileron Adjustment/1(alpha)
  [beta_deg] -> Aileron Adjustment/2(beta)
  [del_lef_deg] -> Aileron Adjustment/3(del_lef)
  [alpha_deg] -> Rudder Adjustment/1(alpha)
  [beta_deg] -> Rudder Adjustment/2(beta)
  [alpha_deg] -> Yaw Rate Damping/1(alpha)
  [del_lef_deg] -> Yaw Rate Damping/2(del_lef)
  [alpha_deg] -> Roll Rate Damping/1(alpha)
  [del_lef_deg] -> Roll Rate Damping/2(del_lef)

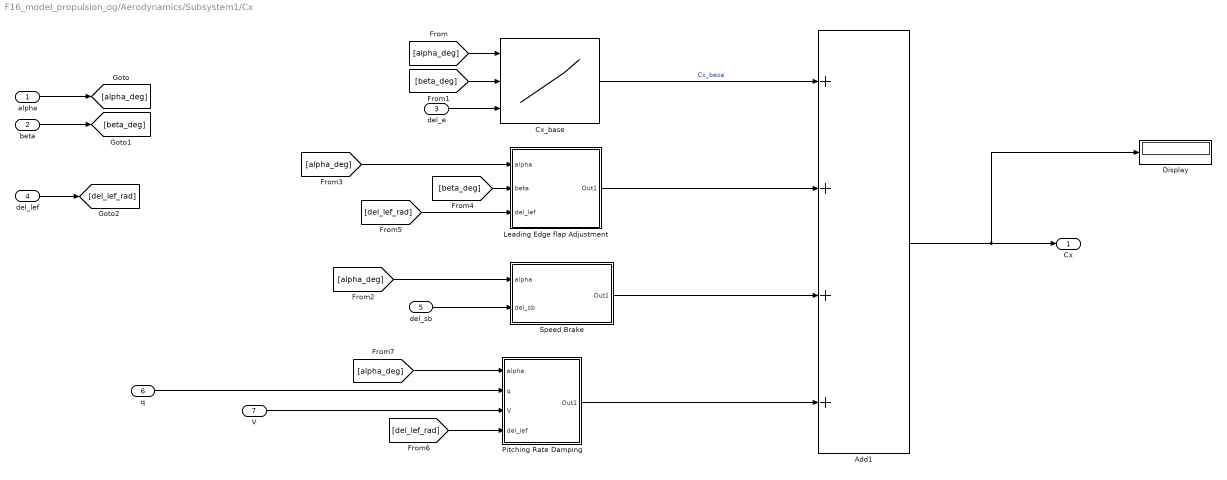
== system F16_model_propulsion_og/Aerodynamics/Subsystem1/Cx ==
  alpha : Inport
  beta : Inport  Port=2
  del_e : Inport  Port=3
  del_lef : Inport  Port=4
  del_sb : Inport  Port=5
  q : Inport  Port=6
  V : Inport  Port=7
  " Cx_base" : Lookup_n-D  NumberOfTableDimensions=3  BreakpointsForDimension1=[-20, -15, -10, -5, 0, 5, 10, 15, 20, 25, 30, 35, 40, 45, 50, 55, 60, 70, 80, 90];  BreakpointsForDimension2=[-30, -25, -20, -15, -10, -8, -6, -4, -2, 0, 2, 4, 6, 8, 10, 15, 20, 25, 30];  BreakpointsForDimension3=[-25, -10, 0, 10, 25];  Table=aero_data.Cx_del_h  InternalRulePriority=Speed  RndMeth=Simplest
      settings: InputPortMap=u0,u1,u2
  Add1 : Sum  Inputs=++++
  Display : Display
  Leading Edge flap Adjustment : Subsystem
  Pitching Rate Damping : Subsystem
  Speed Brake : Subsystem
  Cx : Outport
  wires:
  del_e/1 -> " Cx_base"/3
  Speed Brake/1(Out1) -> Add1/3
  " Cx_base"/1 -> Add1/1  "Cx_base"
  Pitching Rate Damping/1(Out1) -> Add1/4
  Leading Edge flap Adjustment/1(Out1) -> Add1/2
  Add1/1 -> Display/1, Cx/1
  del_sb/1 -> Speed Brake/2(del_sb)
  q/1 -> Pitching Rate Damping/2(q)
  V/1 -> Pitching Rate Damping/3(V)
  alpha/1 -> [alpha_deg]
  beta/1 -> [beta_deg]
  [alpha_deg] -> " Cx_base"/1
  [beta_deg] -> " Cx_base"/2
  del_lef/1 -> [del_lef_rad]
  [alpha_deg] -> Speed Brake/1(alpha)
  [alpha_deg] -> Leading Edge flap Adjustment/1(alpha)
  [beta_deg] -> Leading Edge flap Adjustment/2(beta)
  [del_lef_rad] -> Leading Edge flap Adjustment/3(del_lef)
  [del_lef_rad] -> Pitching Rate Damping/4(del_lef)
  [alpha_deg] -> Pitching Rate Damping/1(alpha)

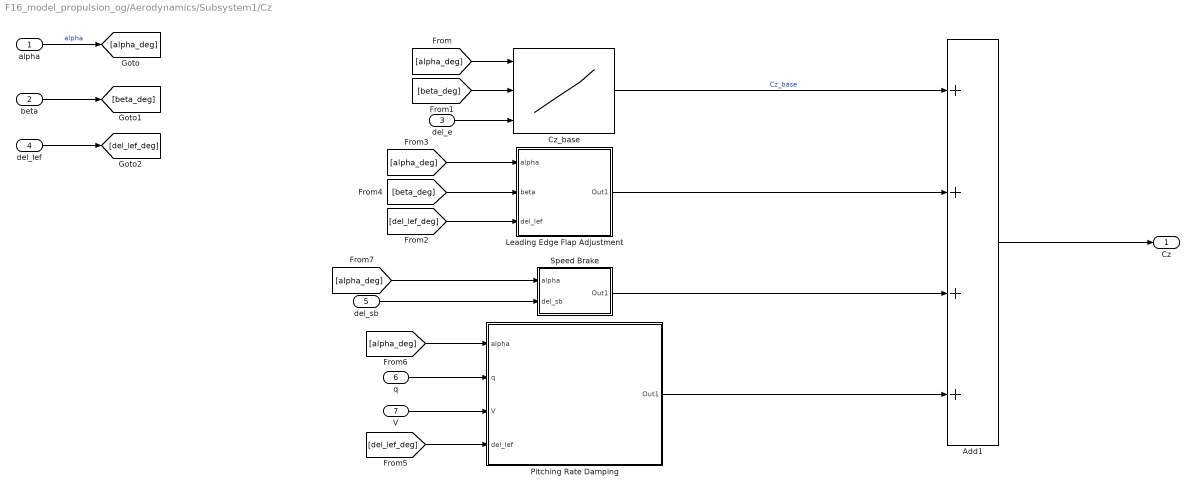
== system F16_model_propulsion_og/Aerodynamics/Subsystem1/Cz ==
  alpha : Inport
  beta : Inport  Port=2
  del_e : Inport  Port=3
  del_lef : Inport  Port=4
  del_sb : Inport  Port=5
  q : Inport  Port=6
  V : Inport  Port=7
  Add1 : Sum  Inputs=++++
  Cz_base : Lookup_n-D  NumberOfTableDimensions=3  BreakpointsForDimension1=[-20, -15, -10, -5, 0, 5, 10, 15, 20, 25, 30, 35, 40, 45, 50, 55, 60, 70, 80, 90];  BreakpointsForDimension2=[-30, -25, -20, -15, -10, -8, -6, -4, -2, 0, 2, 4, 6, 8, 10, 15, 20, 25, 30];  BreakpointsForDimension3=[-25, -10, 0, 10, 25];  Table=aero_data.Cz_del_h  InternalRulePriority=Speed  RndMeth=Simplest
      settings: InputPortMap=u0,u1,u2
  Leading Edge Flap Adjustment : Subsystem
  Pitching Rate Damping : Subsystem
  Speed Brake : Subsystem
  Cz : Outport
  wires:
  del_e/1 -> Cz_base/3
  Speed Brake/1(Out1) -> Add1/3
  Cz_base/1 -> Add1/1  "Cz_base"
  Pitching Rate Damping/1(Out1) -> Add1/4
  Leading Edge Flap Adjustment/1(Out1) -> Add1/2
  Add1/1 -> Cz/1
  del_sb/1 -> Speed Brake/2(del_sb)
  q/1 -> Pitching Rate Damping/2(q)
  V/1 -> Pitching Rate Damping/3(V)
  alpha/1 -> [alpha_deg]  "alpha"
  beta/1 -> [beta_deg]
  [alpha_deg] -> Cz_base/1
  [beta_deg] -> Cz_base/2
  del_lef/1 -> [del_lef_deg]
  [del_lef_deg] -> Leading Edge Flap Adjustment/3(del_lef)
  [alpha_deg] -> Leading Edge Flap Adjustment/1(alpha)
  [beta_deg] -> Leading Edge Flap Adjustment/2(beta)
  [del_lef_deg] -> Pitching Rate Damping/4(del_lef)
  [alpha_deg] -> Pitching Rate Damping/1(alpha)
  [alpha_deg] -> Speed Brake/1(alpha)

== system F16_model_propulsion_og/EqM/EulerAngles/Rotation Matrix ==
  note: LBE
  EulerAngles_rad : Inport
  Math Function : Math  Operator=transpose  SignedPower=on
  Mux : Mux  Inputs=2
  Mux2 : Mux  Inputs=9
  Reshape : Reshape  OutputDimensionality=Customize  OutputDimensions=[3,3]
  Trigonometric Function : Trigonometry  Operator=sincos
  phidot_radps1 : Fcn  Expr=u(1)*u(2)*u(6) - u(4)*u(3)
  phidot_radps2 : Fcn  Expr=u(5)*u(6)
  phidot_radps3 : Fcn  Expr=u(6)*u(2)*u(4) + u(1)*u(3)
  phidot_radps4 : Fcn  Expr=u(5)*u(3)
  phidot_radps5 : Fcn  Expr=u(1)*u(2)*u(3) + u(4)*u(6)
  phidot_radps6 : Fcn  Expr=u(4)*u(2)*u(3) -u(1)*u(6)
  phidot_radps7 : Fcn  Expr=-u(2)
  phidot_radps8 : Fcn  Expr=u(1)*u(5)
  phidot_radps9 : Fcn  Expr=u(4)*u(5)
  LBE : Outport
  wires:
  phidot_radps3/1 -> Mux2/3
  phidot_radps9/1 -> Mux2/9
  phidot_radps6/1 -> Mux2/6
  Mux2/1 -> Reshape/1
  phidot_radps5/1 -> Mux2/5
  Trigonometric Function/1 -> Mux/1
  phidot_radps8/1 -> Mux2/8
  Mux/1 -> phidot_radps3/1, phidot_radps1/1, phidot_radps2/1, phidot_radps9/1, phidot_radps8/1, phidot_radps7/1, phidot_radps6/1, phidot_radps5/1, phidot_radps4/1
  EulerAngles_rad/1 -> Trigonometric Function/1
  phidot_radps1/1 -> Mux2/2
  phidot_radps2/1 -> Mux2/1
  Math Function/1 -> LBE/1
  phidot_radps7/1 -> Mux2/7
  Trigonometric Function/2 -> Mux/2
  phidot_radps4/1 -> Mux2/4
  Reshape/1 -> Math Function/1

== system F16_model_propulsion_og/EqM/EulerAngles/Subsystem ==
  "BodyRates_radps " : Inport
  EulerAngles_rad : Inport  Port=2
  Abs : Abs  SaturateOnIntegerOverflow=off
  Constant : Constant  Value=0.001
  Demux1 : Demux  Outputs=3
  Mux : Mux  Inputs=3
  Mux2 : Mux  Inputs=3
  Mux3 : Mux  Inputs=3
  Product : Product
  Relay : Relay  OnSwitchValue=.001  OffSwitchValue=0  OnOutputValue=0  OffOutputValue=1
  Sign : Signum
  Switch : Switch  Criteria=u2 > Threshold  Threshold=0.5  SaturateOnIntegerOverflow=off  InputSameDT=off
  Trigonometric Function : Trigonometry  Operator=sincos
  phidot_radps2 : Fcn  Expr=u(1)+u(2)*u(4)*(u(5)/u(8))+u(3)*u(7)*(u(5)/u(8))
  psidot_radps2 : Fcn  Expr=(u(2)*u(4)+u(3)*u(7))/u(8)
  thetadot_radps2 : Fcn  Expr=u(2)*u(7)-u(3)*u(4)
  EulerRates_radsps2 : Outport
  wires:
  Demux1/2 -> Sign/1, Abs/1, Switch/3
  Mux2/1 -> Mux/3
  phidot_radps2/1 -> Mux3/1
  Relay/1 -> Switch/2
  Demux1/3 -> Mux2/3
  Trigonometric Function/2 -> Demux1/1
  Mux/1 -> phidot_radps2/1, thetadot_radps2/1, psidot_radps2/1
  Demux1/1 -> Mux2/1
  Abs/1 -> Relay/1
  psidot_radps2/1 -> Mux3/3
  Sign/1 -> Product/2
  Switch/1 -> Mux2/2
  Product/1 -> Switch/1
  Mux3/1 -> EulerRates_radsps2/1
  EulerAngles_rad/1 -> Trigonometric Function/1
  thetadot_radps2/1 -> Mux3/2
  Trigonometric Function/1 -> Mux/2
  Constant/1 -> Product/1
  "BodyRates_radps "/1 -> Mux/1

== system F16_model_propulsion_og/Aerodynamics/Subsystem1/C_y/Aileron Adjustment ==
  "Cy(alpha, beta)" : Inport
  alpha : Inport  Port=2
  beta : Inport  Port=3
  del_a : Inport  Port=4
  del_lef : Inport  Port=5
  Add1 : Sum
  Cy_del_a_20 : Lookup_n-D  BreakpointsForDimension1=[-20, -15, -10, -5, 0, 5, 10, 15, 20, 25, 30, 35, 40, 45, 50, 55, 60, 70, 80, 90];  BreakpointsForDimension2=[-30, -25, -20, -15, -10, -8, -6, -4, -2, 0, 2, 4, 6, 8, 10, 15, 20, 25, 30];  Table=aero_data.Cy_del_a_20  InternalRulePriority=Speed  RndMeth=Simplest
      settings: InputPortMap=u0,u1
  Multiply1 : Gain  Gain=0.05
  Product2 : Product
  Subtract1 : Sum  Inputs=-+
  del_Cy_del_a_20*(1-del_lef/25) : Subsystem
  Out1 : Outport
  wires:
  beta/1 -> Cy_del_a_20/2, del_Cy_del_a_20*(1-del_lef/25)/2(beta)
  Multiply1/1 -> Product2/2
  Add1/1 -> Product2/1
  Subtract1/1 -> Add1/1
  del_a/1 -> Multiply1/1
  Cy_del_a_20/1 -> Subtract1/2  "Cy_del_a_20"
  del_Cy_del_a_20*(1-del_lef/25)/1(Out1) -> Add1/2
  del_lef/1 -> del_Cy_del_a_20*(1-del_lef/25)/3(del_lef)
  Product2/1 -> Out1/1
  alpha/1 -> del_Cy_del_a_20*(1-del_lef/25)/1(alpha), Cy_del_a_20/1
  "Cy(alpha, beta)"/1 -> Subtract1/1

== system F16_model_propulsion_og/Aerodynamics/Subsystem1/C_y/Flap Adjustment ==
  "Cy(alpha, beta)" : Inport
  alpha : Inport  Port=2
  beta : Inport  Port=3
  del_lef : Inport  Port=4
  1-del_lef/25 : Subsystem
  Cy_lef : Lookup_n-D  BreakpointsForDimension1=[-20, -15, -10, -5, 0, 5, 10, 15, 20, 25, 30, 35, 40, 45];  BreakpointsForDimension2=[-30, -25, -20, -15, -10, -8, -6, -4, -2, 0, 2, 4, 6, 8, 10, 15, 20, 25, 30];  Table=aero_data.Cy_lef  InternalRulePriority=Speed  RndMeth=Simplest
      settings: InputPortMap=u0,u1
  Product3 : Product
  Subtract2 : Sum  Inputs=+-
  Out1 : Outport
  wires:
  "Cy(alpha, beta)"/1 -> Subtract2/2
  1-del_lef/25/1(1 - del_lef/25) -> Product3/2
  del_lef/1 -> 1-del_lef/25/1(del_lef1)
  Cy_lef/1 -> Subtract2/1  "Cy_lef"
  Subtract2/1 -> Product3/1
  alpha/1 -> Cy_lef/1
  beta/1 -> Cy_lef/2
  Product3/1 -> Out1/1

== system F16_model_propulsion_og/Aerodynamics/Subsystem1/C_y/Roll Rate Damping ==
  alpha : Inport
  del_lef : Inport  Port=2
  p : Inport  Port=3
  Add : Sum
  Constant : Constant
  Constant1 : Constant  Value=25
  Cy_p : Lookup_n-D  NumberOfTableDimensions=1  BreakpointsForDimension1=[-20, -15, -10, -5, 0, 5, 10, 15, 20, 25, 30, 35, 40, 45, 50, 55, 60, 70, 80, 90];  Table=aero_data.Cy_p  InternalRulePriority=Speed  RndMeth=Simplest
  Divide : Product  Inputs=*/
  Product : Product
  Product1 : Product
  Subtract : Sum  Inputs=+-
  del_Cy_p_lef : Lookup_n-D  NumberOfTableDimensions=1  BreakpointsForDimension1=[-20, -15, -10, -5, 0, 5, 10, 15, 20, 25, 30, 35, 40, 45];  Table=aero_data.del_Cy_p_lef  InternalRulePriority=Speed  RndMeth=Simplest
  Out1 : Outport
  wires:
  alpha/1 -> del_Cy_p_lef/1, Cy_p/1
  del_Cy_p_lef/1 -> Product/1  "del_Cy_p_lef"
  Cy_p/1 -> Add/1
  del_lef/1 -> Divide/1
  Constant1/1 -> Divide/2
  Constant/1 -> Subtract/1
  Divide/1 -> Subtract/2
  Subtract/1 -> Product/2  "1 - del_lef/25"
  Product/1 -> Add/2
  Add/1 -> Product1/1
  p/1 -> Product1/2
  Product1/1 -> Out1/1

== system F16_model_propulsion_og/Aerodynamics/Subsystem1/C_y/Rudder Adjustment ==
  "Cy(alpha, beta)" : Inport
  alpha : Inport  Port=2
  beta : Inport  Port=3
  del_r : Inport  Port=4
  Cy_del_r_30 : Lookup_n-D  BreakpointsForDimension1=[-20, -15, -10, -5, 0, 5, 10, 15, 20, 25, 30, 35, 40, 45, 50, 55, 60, 70, 80, 90];  BreakpointsForDimension2=[-30, -25, -20, -15, -10, -8, -6, -4, -2, 0, 2, 4, 6, 8, 10, 15, 20, 25, 30];  Table=aero_data.Cy_r_del_r_30  InternalRulePriority=Speed  RndMeth=Simplest
      settings: InputPortMap=u0,u1
  Product1 : Product
  Subtract : Sum  Inputs=+-
  Out1 : Outport
  wires:
  "Cy(alpha, beta)"/1 -> Subtract/2
  del_r/1 -> Product1/1
  Subtract/1 -> Product1/2
  Cy_del_r_30/1 -> Subtract/1  "Cy_del_r_30"
  alpha/1 -> Cy_del_r_30/1
  beta/1 -> Cy_del_r_30/2
  Product1/1 -> Out1/1

== system F16_model_propulsion_og/Aerodynamics/Subsystem1/C_y/Yaw Rate Damping ==
  alpha : Inport
  del_lef : Inport  Port=2
  r : Inport  Port=3
  Add : Sum
  Constant : Constant
  Constant1 : Constant  Value=25
  Cy_r : Lookup_n-D  NumberOfTableDimensions=1  BreakpointsForDimension1=[-20, -15, -10, -5, 0, 5, 10, 15, 20, 25, 30, 35, 40, 45, 50, 55, 60, 70, 80, 90];  Table=aero_data.Cy_r  InternalRulePriority=Speed  RndMeth=Simplest
  Divide : Product  Inputs=*/
  Product : Product
  Product1 : Product
  Subtract : Sum  Inputs=+-
  del_Cy_r_lef : Lookup_n-D  NumberOfTableDimensions=1  BreakpointsForDimension1=[-20, -15, -10, -5, 0, 5, 10, 15, 20, 25, 30, 35, 40, 45];  Table=aero_data.del_Cy_r_lef  InternalRulePriority=Speed  RndMeth=Simplest
  Out1 : Outport
  wires:
  Cy_r/1 -> Add/1
  alpha/1 -> del_Cy_r_lef/1, Cy_r/1
  del_Cy_r_lef/1 -> Product/1
  del_lef/1 -> Divide/1
  Divide/1 -> Subtract/2
  Subtract/1 -> Product/2  "1 - del_lef/25"
  Constant/1 -> Subtract/1
  Constant1/1 -> Divide/2
  Product/1 -> Add/2
  Add/1 -> Product1/1
  r/1 -> Product1/2
  Product1/1 -> Out1/1
